simulink model "stanley_control"  (R2021a)
settings: Solver=FixedStepAuto  StartTime=0.0  StopTime=Ts  FixedStep=0.1  RelTol=1e-3
InitFcn:
  | Stanley_control_init
StopFcn:
  | Lateral_plot
values from neighbouring files (symbols this model uses):
  vRef = 10    [Stanley_control_init.m]
libraries: simulink_extras x1, drivingvehiclecontroller x1, autolibshared x1
settings Model: Creator=User  LastModifiedBy=User

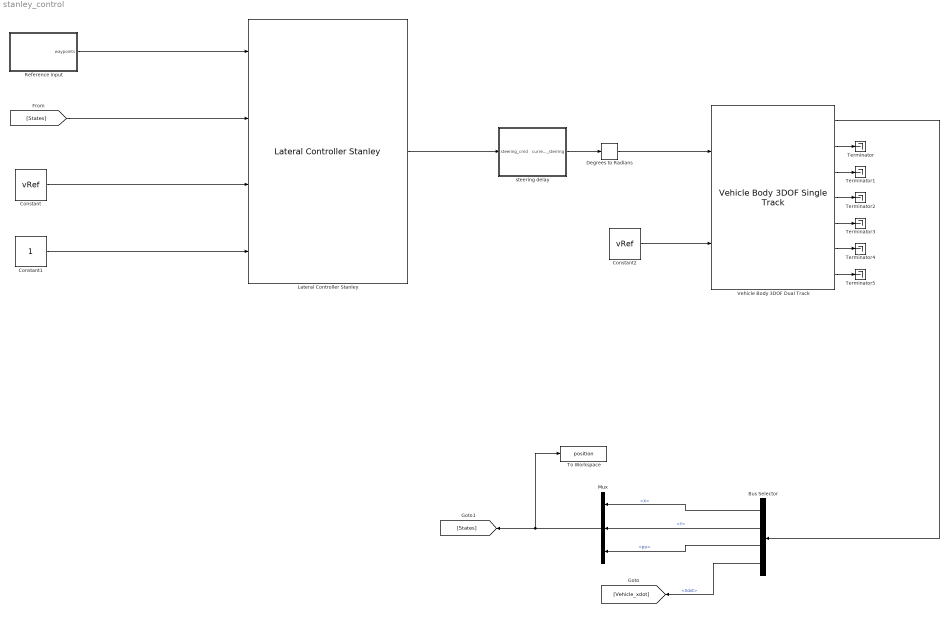
== system stanley_control ==
  Bus Selector : BusSelector  OutputSignals=InertFrm.Cg.Disp.X,InertFrm.Cg.Disp.Y,InertFrm.Cg.Ang.psi,InertFrm.Cg.Vel.Xdot
  Constant : Constant  Value=vRef
  Constant1 : Constant
  Constant2 : Constant  Value=vRef
  Degrees to Radians : simulink_extras/Transformations/Degrees to Radians
  Lateral Controller Stanley : drivingvehiclecontroller/Lateral Controller Stanley  ModelType=Kinematic bicycle model  PositionGainF=K  PositionGainR=1  YawRateGain=0.2  DelayGain=0.2  VehicleMass=1575  Lf=1.2  Lr=1.6  TireStiffness=19000  Wheelbase=L  MaxSteeringAngle=35
      settings: SourceProductBaseCode=DR
  Mux : Mux  Inputs=3
  Reference input : Subsystem
  Terminator{,1..5} (6 alike) : Terminator
  To Workspace : ToWorkspace  VariableName=position  SaveFormat=Timeseries  SampleTime=-1
  Vehicle Body 3DOF Dual Track : autolibshared/Vehicle Body 3DOF Single Track  trackMode=Dual  inputMode=External longitudinal velocity  frontSteerMode=on  rearSteerMode=off  windMode=off  muMode=off  extFMode=off  extMMode=off  htchFMode=off  htchMMode=off  extXo=off  extpsio=off  extxdoto=off  extro=off  extYo=off  extTamb=off  extydoto=off  aMode=2  NF=2  NR=2  m=1575  a=1.2  b=1.6  h=0.35  dh=1  hh=0.2  X_o=X_0  xdot_o=0  CalphaMode=off  sigmaMode=on  d=0  hl=0  w=[1.4,1.4]  Cy_f=19e3  Cy_r=20e3  sigma_f=.1  sigma_r=.1  alpha_f_brk=[-.1 .1]  Cy_f_data=[-9e3 9e3]  alpha_r_brk=[-.1 .1]  Cy_r_data=[-9e3 9e3]  Y_o=Y_0  ydot_o=0  Izz=4000  psi_o=0  r_o=psi_0  Af=2  Cd=.3  Cl=.1  Cpm=.1  beta_w=[0:0.01:0.3]  Cs=[0:0.03:0.9]  Cym=[0:0.01:0.3]  Pabs=101325  Tair=273  g=9.81  mu=1  xdot_tol=.01  Fznom=5000  Fxtire_sat=7e4  Fytire_sat=7e4  longOff=0  latOff=0  vertOff=0  wrapAng=off
      settings: SourceProductBaseCode=PW,DR,MT,UV,VE
  steering delay : Subsystem
  wires:
  Reference input/1(waypoints) -> Lateral Controller Stanley/1
  Constant/1 -> Lateral Controller Stanley/3
  Constant1/1 -> Lateral Controller Stanley/4
  Lateral Controller Stanley/1 -> steering delay/1(steering_cmd)
  steering delay/1("current_sterring ") -> Degrees to Radians/1
  Constant2/1 -> Vehicle Body 3DOF Dual Track/2
  Degrees to Radians/1 -> Vehicle Body 3DOF Dual Track/1
  Vehicle Body 3DOF Dual Track/2 -> Terminator/1
  Vehicle Body 3DOF Dual Track/3 -> Terminator1/1
  Vehicle Body 3DOF Dual Track/4 -> Terminator2/1
  Vehicle Body 3DOF Dual Track/5 -> Terminator3/1
  Vehicle Body 3DOF Dual Track/6 -> Terminator4/1
  Vehicle Body 3DOF Dual Track/7 -> Terminator5/1
  Vehicle Body 3DOF Dual Track/1 -> Bus Selector/1
  Bus Selector/1 -> Mux/1  "<X>"
  Bus Selector/2 -> Mux/2  "<Y>"
  Bus Selector/3 -> Mux/3  "<psi>"
  Bus Selector/4 -> [Vehicle_xdot]  "<Xdot>"
  Mux/1 -> [States], To Workspace/1
  [States] -> Lateral Controller Stanley/2

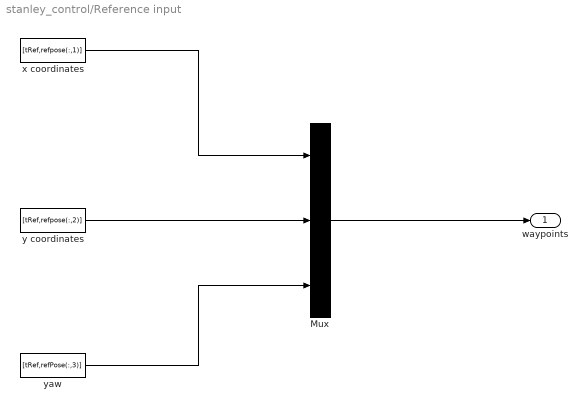
== system stanley_control/Reference input ==
  Mux : Mux  Inputs=3
  x coordinates : FromWorkspace  VariableName=[tRef,refpose(:,1)]  SampleTime=0.1
  y coordinates : FromWorkspace  VariableName=[tRef,refpose(:,2)]  SampleTime=0.1
  yaw : FromWorkspace  VariableName=[tRef,refPose(:,3)]  SampleTime=0.1
  waypoints : Outport
  wires:
  y coordinates/1 -> Mux/2
  x coordinates/1 -> Mux/1
  yaw/1 -> Mux/3
  Mux/1 -> waypoints/1

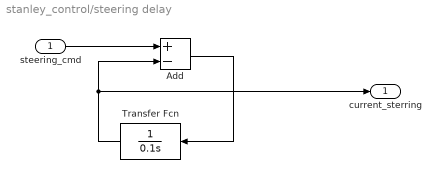
== system stanley_control/steering delay ==
  steering_cmd : Inport
  Add : Sum  Inputs=+-
  Transfer Fcn : TransferFcn  Denominator=[0.1 0]
  "current_sterring " : Outport
  wires:
  steering_cmd/1 -> Add/1
  Transfer Fcn/1 -> "current_sterring "/1, Add/2
  Add/1 -> Transfer Fcn/1
